simulink model "gz_zitai"  (Simulink 6.2)
settings: Solver=ode3  StartTime=0.0  StopTime=5  FixedStep=0.005  RelTol=1e-3
values from neighbouring files (symbols this model uses):
  b11 = -0.05*Q*serf*L*L/jx/v    [sim_3dof.m]
  b17 = (gz3(ma_cnt,alpha_cnt)-gz1(ma_cnt,alpha_cnt))/(1/57.3)/jx*Q*serf*L    [sim_3dof.m]
settings Model: LastModifiedBy=wangjsh
settings DebuggingCC: SolverPrmCheckMsg=warning

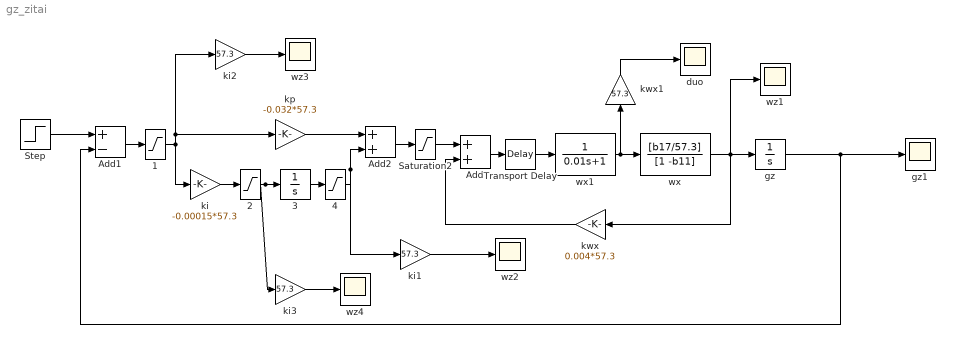
== system gz_zitai ==
  1 : Saturate  UpperLimit=300/57.3  LowerLimit=-300/57.3  LinearizeAsGain=off
  2 : Saturate  UpperLimit=100/57.3  LowerLimit=-100/57.3  LinearizeAsGain=off
  3 : Integrator
  4 : Saturate  UpperLimit=130/57.3  LowerLimit=-130/57.3  LinearizeAsGain=off
  Add : Sum  OutScaling=2^-10
  Add1 : Sum  Inputs=+-  OutScaling=2^-10
  Add2 : Sum  OutScaling=2^-10
  Saturation2 : Saturate  UpperLimit=10/57.3  LowerLimit=-10/57.3
  Step : Step  Time=0  SampleTime=0
  Transport Delay : TransportDelay  DelayTime=0.0
  duo : Scope
      settings: SaveName=ScopeData2
  gz : Integrator
  gz1 : Scope
      settings: TimeRange=3
  ki : Gain  Gain=-0.00015*57.3
  ki1 : Gain  Gain=57.3
  ki2 : Gain  Gain=57.3
  ki3 : Gain  Gain=57.3
  kp : Gain  Gain=-0.032*57.3
  kwx : Gain  Orientation=left  Gain=0.004*57.3
  kwx1 : Gain  Orientation=up  Gain=57.3
  wx : TransferFcn  Numerator=[b17/57.3]  Denominator=[1 -b11]
  wx1 : TransferFcn  Denominator=[0.01 1]
  wz{1..4} (4 alike) : Scope
      wz2 settings: SaveName=ScopeData3
      wz3 settings: SaveName=ScopeData4
      wz4 settings: SaveName=ScopeData5
  wires:
  wx/1 -> gz/1, kwx/1, wz1/1
  Add/1 -> Transport Delay/1
  kwx/1 -> Add/2
  gz/1 -> gz1/1, Add1/2
  Step/1 -> Add1/1
  Add1/1 -> 1/1
  kp/1 -> Add2/1
  ki/1 -> 2/1
  Transport Delay/1 -> wx1/1
  Add2/1 -> Saturation2/1
  3/1 -> 4/1
  1/1 -> ki/1, kp/1, ki2/1
  kwx1/1 -> duo/1
  2/1 -> 3/1, ki3/1
  4/1 -> Add2/2, ki1/1
  wx1/1 -> wx/1, kwx1/1
  Saturation2/1 -> Add/1
  ki1/1 -> wz2/1
  ki2/1 -> wz3/1
  ki3/1 -> wz4/1
